simulink model "Model"  (R2022b)
settings: Solver=VariableStepAuto  StartTime=0.0  StopTime=10  FixedStep=1e-3  RelTol=1e-3
InitFcn:
  | ModelParameters
values from neighbouring files (symbols this model uses):
  ref_set = [1.5,-1.5,1,0]    [ModelParameters.m]
  X_init = [1,1,0,  0,0,0,  0,0,1, 0,0,0]    [ModelParameters.m]
settings Model: Creator=samuel  LastModifiedBy=sebas
settings SolverCC: ZeroCrossControl=DisableAll  AlgebraicLoopSolver=TrustRegion
settings DebuggingCC: UnconnectedInputMsg=warning  UnconnectedOutputMsg=warning  UnconnectedLineMsg=warning  SFMachineParentedDataDiag=warning  UnderSpecifiedDimensionMsg=warning  ArithmeticOperatorsInVariantConditions=warning
settings ModelReferenceCC: EnableRefExpFcnMdlSchedulingChecks=on
settings SFSimCC: CustomCodeUndefinedFunction=UseInterfaceOnly

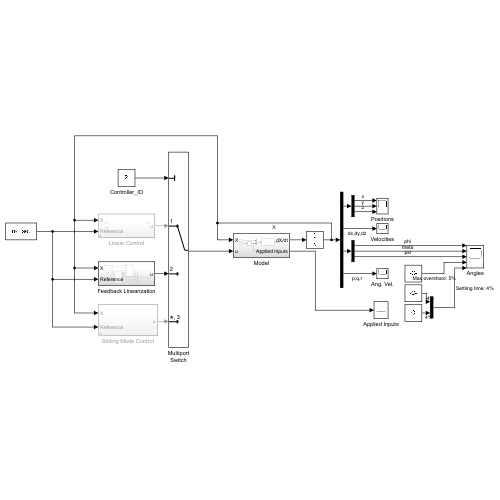
[thumbnail: Simulink's stored preview of the top-level diagram]
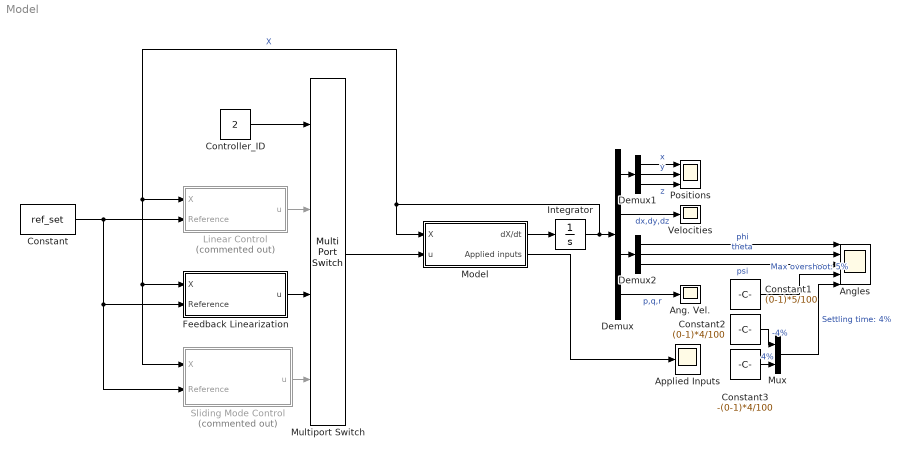
== system Model ==
  Ang. Vel. : Scope
  Angles : Scope  NumInputPorts=5
  "Applied Inputs " : Scope
  Constant : Constant  Value=ref_set
  Constant1 : Constant  Value=(0-1)*5/100
  Constant2 : Constant  Value=(0-1)*4/100
  Constant3 : Constant  Value=-(0-1)*4/100
  Controller_ID : Constant  Value=2
  Demux : Demux  Outputs=[3,3,3,3]
  Demux1 : Demux  Outputs=3
  Demux2 : Demux  Outputs=3
  Feedback Linearization : Subsystem
  Integrator : Integrator  InitialCondition=X_init
  Linear Control : Subsystem  Commented=on
  Model : Subsystem
  Multiport Switch : MultiPortSwitch  DataPortOrder=Specify indices  SaturateOnIntegerOverflow=off  InputSameDT=off
  Mux : Mux  Inputs=2
  Positions : Scope  NumInputPorts=3
  Sliding Mode Control : Subsystem  Commented=on
  Velocities : Scope
  wires:
  Model/1(dX/dt) -> Integrator/1
  Integrator/1 -> Demux/1, Sliding Mode Control/1(X), Feedback Linearization/1(X), Linear Control/1(X), Model/1(X)  "X"
  Constant/1 -> Linear Control/2(Reference), Feedback Linearization/2(Reference), Sliding Mode Control/2(Reference)
  Demux/2 -> Velocities/1  "dx,dy,dz"
  Demux/4 -> Ang. Vel./1  "p,q,r"
  Multiport Switch/1 -> Model/2(u)
  Controller_ID/1 -> Multiport Switch/1
  Feedback Linearization/1(u) -> Multiport Switch/3
  Linear Control/1(u) -> Multiport Switch/2
  Sliding Mode Control/1(u) -> Multiport Switch/4
  Model/2(Applied inputs) -> "Applied Inputs "/1
  Demux/1 -> Demux1/1
  Demux1/1 -> Positions/1  "x"
  Demux1/2 -> Positions/2  "y"
  Demux1/3 -> Positions/3  "z"
  Demux/3 -> Demux2/1
  Demux2/1 -> Angles/1  "phi"
  Demux2/2 -> Angles/2  "theta"
  Demux2/3 -> Angles/3  "psi"
  Constant1/1 -> Angles/4  "Max overshoot: 5%"
  Constant3/1 -> Mux/2  "4%"
  Constant2/1 -> Mux/1  "-4%"
  Mux/1 -> Angles/5  "Settling time: 4%"

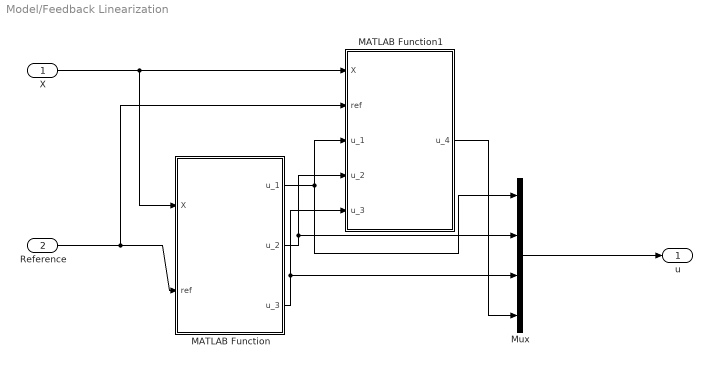
== system Model/Feedback Linearization ==
  X : Inport
  Reference : Inport  Port=2
  MATLAB Function : MATLAB Function  TreatAsAtomicUnit=on
  MATLAB Function1 : MATLAB Function  TreatAsAtomicUnit=on
  Mux : Mux
  u : Outport
  wires:
  MATLAB Function/2(u_2) -> Mux/2, MATLAB Function1/4(u_2)
  Mux/1 -> u/1
  MATLAB Function1/1(u_4) -> Mux/4
  Reference/1 -> MATLAB Function/2(ref), MATLAB Function1/2(ref)
  X/1 -> MATLAB Function/1(X), MATLAB Function1/1(X)
  MATLAB Function/3(u_3) -> MATLAB Function1/5(u_3), Mux/3
  MATLAB Function/1(u_1) -> MATLAB Function1/3(u_1), Mux/1

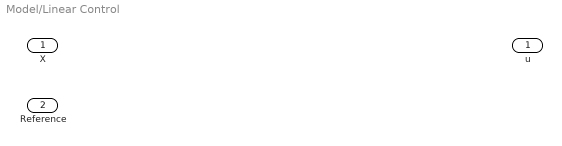
== system Model/Linear Control ==
  X : Inport
  Reference : Inport  Port=2
  u : Outport

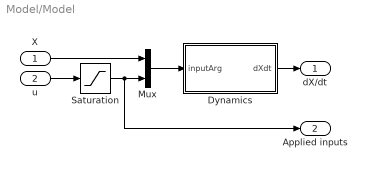
== system Model/Model ==
  X : Inport
  u : Inport  Port=2
  Dynamics : MATLAB Function  TreatAsAtomicUnit=on
  Mux : Mux  Inputs=2
  Saturation : Saturate  UpperLimit=10  LowerLimit=-10
  dX/dt : Outport
  Applied inputs : Outport  Port=2
  wires:
  X/1 -> Mux/1
  u/1 -> Saturation/1
  Dynamics/1(dXdt) -> dX/dt/1
  Mux/1 -> Dynamics/1(inputArg)
  Saturation/1 -> Applied inputs/1, Mux/2

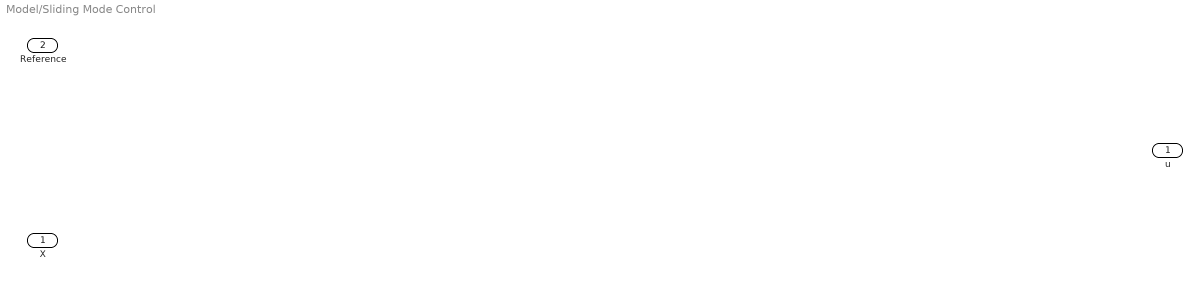
== system Model/Sliding Mode Control ==
  X : Inport
  Reference : Inport  Port=2
  u : Outport  VectorParamsAs1DForOutWhenUnconnected=off

== matlab function Model/Feedback Linearization/MATLAB Function ==
  data: X input; u_1 output; ref input; u_2 output; u_3 output
function [u_1,u_2,u_3] = xyzController(X,ref)

% Compute x and y errors
e_x = X(1)-ref(1);
e_y = X(2)-ref(2);
e_z = X(3)-ref(3);

psi = X(9);

% Rotate into body frame (approximate, only accounts for yaw)
e_x_B = e_x*cos(psi) + e_y*sin(psi);
e_y_B = -e_x*sin(psi) + e_y*cos(psi);

v_x = X(4)*cos(psi) +X(5)*sin(psi);
v_y = -X(4)*sin(psi) + X(5)*cos(psi);
v_z = X(6);

% Compute inputs using feedback
kp_z = -5;
kd_z = -1;

kp_xy = -1;
kd_xy = -1.6;

kp_rot = -5;
kd_rot = -1;

m  = 28e-3;
g = 9.8;
% 
u_1 = m*g + kp_z*e_z + kd_z*v_z;
u_2 = -kp_xy*e_y_B - kd_xy*v_y + kp_rot*X(7) + kd_rot*X(10);
u_3 = kp_xy*e_x_B + kd_xy*v_x + kp_rot*X(8) + kd_rot*X(11);

end

== matlab function Model/Dynamics ==
  data: inputArg input; dXdt output
function dXdt  = nlmodel(inputArg)
%NLMODEL Compute full state derivative
%   Using non-linear model

%% Parse input

nStates = 12;
nInputs = 4;
% assert(min(size(inputArg) == [1 (nStates + nInputs)]));
X = inputArg(1:nStates);
u = inputArg(nStates + 1:nStates + nInputs);
dXdt = zeros(nStates, 1);

%[x y z dx dy dz theta phi psi p q r] = X;
x       = X(1);
y       = X(2);
z       = X(3);
dx      = X(4);
dy      = X(5);
dz      = X(6);
phi     = X(7);
theta   = X(8);
psi     = X(9);
p       = X(10);
q       = X(11);
r       = X(12);

%% Model parameters

m  = 28e-3;
Ix = 16.57e-6;
Iy = 29.51e-6;
Iz = 29.26e-6;
% 
% m  = 0.65;
% Ix = 7.5e-3;
% Iy = 7.5e-3;
% Iz = 1.3e-2;

Kx = 0.01;
Ky = 0.01;
Kz = 0.01;
Kp = 1e-5;
Kq = 1e-5;
Kr = 1e-5 ;
g  = 9.8;


%% Equations of motion

% 1st derivatives of the position
dXdt(1:3) = X(4:6);

% Eq. 3
dXdt(4) = (1/m) * ((cos(phi)*sin(theta)*cos(psi) + sin(phi)*sin(psi))*u(1) - Kx*dx);
dXdt(5) = (1/m) * ((cos(phi)*sin(theta)*sin(psi) - sin(phi)*cos(psi))*u(1) - Ky*dy);
dXdt(6) = (1/m) * (cos(phi)*cos(theta)*u(1) - m*g - Kz*dz);

% Eq. 1
dXdt(7) = p + q*sin(phi)*tan(theta) +  r*cos(phi)*tan(theta);
dXdt(8) = q*cos(phi) - r*sin(phi);
dXdt(9) = q*sin(phi)/cos(theta) + r*cos(phi)/cos(theta);
         
% Eq. 4
dXdt(10) = (1/Ix)*((Iy-Iz)*q*r + u(2) - Kp*p);
dXdt(11) = (1/Iy)*((Iz-Ix)*p*r + u(3) - Kq*q);
dXdt(12) = (1/Iz)*((Ix-Iy)*p*q + u(4) - Kr*r);

%% Check output dimensions

assert(min(size(dXdt) == [nStates, 1]));
end

== matlab function Model/Feedback Linearization/MATLAB Function1 ==
  data: X input; u_4 output; ref input; u_1 input; u_2 input; u_3 input
function u_4  = yawController(X,ref,u_1,u_2,u_3)
% control params
K_1 = 4; % P
K_2 = 3; % D
% system params
Ix = 16.57e-6;
Iy = 29.51e-6;
Iz = 29.26e-6;
kq = 10e-6;
kr = 10e-6;

den = cos(X(7))/(Iz * cos(X(8)));
num = (1 / Iy) * ((Iz - Ix) * X(10) * X(12) + u_3 - kq * X(11)) * sin(X(7)) / cos(X(8)) + ...
    (X(11) * cos(X(7)) / cos(X(8)) - X(12) * sin(X(7)) / cos(X(8))) * (X(10) + X(11) * sin(X(7)) * tan(X(8)) + X(12) * cos(X(7)) * tan(X(8))) + ...
    (X(11) * sin(X(7)) * sin(X(8)) + X(12) * cos(X(7)) * sin(X(8))) * (X(11) * cos(X(7)) - X(12) * sin(X(7))) * (1 / (cos(X(8))) ^ 2) + ...
    (1 / Iz) * ((Ix - Iy) * X(10) * X(11) - kr * X(12)) * cos(X(7)) / cos(X(8));

psi_dot = X(11) * sin(X(7)) / cos(X(8)) + X(12) * cos(X(7)) / cos(X(8));
u_4 = (1 / den) * (- num - K_1 * (X(9) - ref(4)) - K_2 * psi_dot);

end
